simulink model "system2020b"  (R2020b)
settings: Solver=VariableStepAuto  StartTime=0.0  StopTime=50  RelTol=1e-3
InitFcn:
  | parametriEgo
values from neighbouring files (symbols this model uses):
  campnormalized = campmag/sqrt(campmag(1)^2+campmag(2)^2+campmag(3)^2)    [parametriEgo.m]
  g = 9.81    [kalman_jacobian.m]    (also in parametriEgo.m = [0; 0; -9.81])
  initial_conditions = [0,0,0*pi/180,0*pi/180,0,0]    [parametriEgo.m]
  k_e_qf = 0.1    [ego_control_gains_sensors.m]
  ki_e_nu_speed = 2.5    [ego_control_gains_sensors.m]
  kp_e_nu_phidot = 7    [ego_control_gains_sensors.m]
  kp_e_nu_speed = 6    [ego_control_gains_sensors.m]
  kp_e_nu_thetadot = 7    [ego_control_gains_sensors.m]
  kp_e_theta = 40    [ego_control_gains_sensors.m]
  l = 0.248    [parametriEgo.m]
  L = 0.379    [parametriEgo.m]
  mb = 21.7+0.536*10+0.381*2    (= 27.822)    [parametriEgo.m]
  mw = 1.6    [parametriEgo.m]
  P0 = 1500*eye(7)    [parametriEgo.m]
  r = 0.13    [parametriEgo.m]
  seedAcc1 = ceil(rand()*10)    [parametriEgo.m]
  seedAcc2 = ceil(rand()*10)    [parametriEgo.m]
  seedGyro1 = ceil(rand()*10)    [parametriEgo.m]
  seedGyro2 = ceil(rand()*10)    [parametriEgo.m]
  tau_max = 11    [parametriEgo.m]
  totAccNoisePower = (accNoiseDens* 10^-6 * 9.8)^2    (= 8.6436e-06)    [parametriEgo.m]
  totGyroNoisePower = (gyroNoiseDens * pi/180)^2    (= 3.04617419787e-06)    [parametriEgo.m]
  Ts = 1/100    (= 0.01)    [parametriEgo.m]
  TsController = 1/100    (= 0.01)    [parametriEgo.m]
  TsGraph = 1/100    (= 0.01)    [parametriEgo.m]
  x0 = zeros(7,1)    [parametriEgo.m]
undefined symbols (not defined in the file or in its folder): alpha
libraries: simulink_extras x45, simulink x10, eeGeneralControl x3
(part 1 of 3)
settings Model: Creator=pcfilm  LastModifiedBy=stefa
settings DebuggingCC: SFMachineParentedDataDiag=error

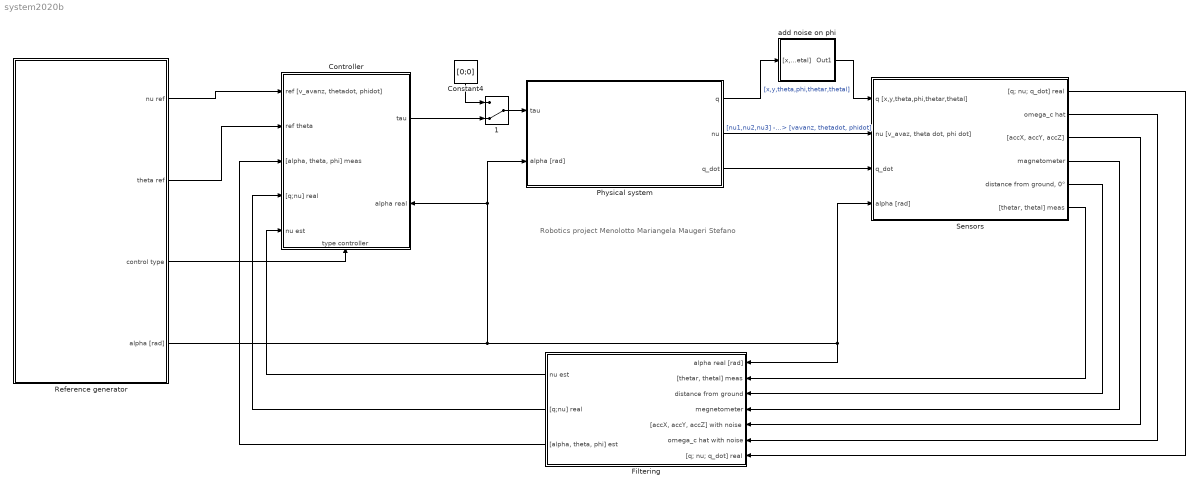
== system system2020b ==
  note: Robotics project
      | Menolotto Mariangela
      | Maugeri Stefano
  " 1" : ManualSwitch  StopFcn=show_results  CurrentSetting=0
  Constant4 : Constant  Value=[0;0]  SampleTime=-1
  Controller : Subsystem
      settings: PortSchema="{\"entries\":[{\"content\":{\"sides\":[{\"content\":{\"connectorIds\":[\"In1\",\"In2\",\"In3\",\"In4\",\"In5\"]},\"type\":\"ConnectorPlacement.EquallySpacedRectSide\",\"uuid\":\"8f36a280-abce-482b-9b97-e189d55cf96d\"},{\"content\":{\"connectorIds\":[\"Out1\",\"In7\"],\"side\":\"RIGHT\"},\"type\":\"ConnectorPlacement.EquallySpacedRectSide\",\"uuid\":\"71f54387-a45a-4e5e-9582-a0f1ed7853f2\"},{\"content\":{\"connectorIds\":[],\"side\":\"TOP\"},\"type\":\"ConnectorPlacement.EquallySpacedRectSide\",\"uuid\":\"bc3039b8-0052-42d5-8d22-75d00eb9e222\"},{\"content\":{\"connectorIds\":[\"In6\"],\"side\":\"BOTTOM\"},\"type\":\"ConnectorPlacement.EquallySpacedRectSide\",\"uuid\":\"65646135-8cf5-4f6c-bd6c-0ad1be6a71b3\"}]},\"type\":\"ConnectorPlacement.EquallySpacedConnector\",\"uuid\":\"29576908-5cc3-45a2-91a3-f3615a274226\"}],\"packageUris\":[\"http://schema.mathworks.com/mf0/Connector/R2020b\"],\"version\":\"1.0\"}"
  Filtering : Subsystem
  Physical system : Subsystem
  Reference generator : Subsystem
  Sensors : Subsystem
  add noise on phi : Subsystem
  wires:
  Constant4/1 -> " 1"/1
  Controller/1(tau) -> " 1"/2
  Physical system/2(nu) -> Sensors/2("nu [v_avaz, theta dot, phi dot]")  "[nu1,nu2,nu3] -> [vavanz, thetadot, phidot]"
  " 1"/1 -> Physical system/1(tau)
  Reference generator/3(control type) -> Controller/6(type controller)
  Reference generator/1(nu ref) -> Controller/1("ref [v_avanz, thetadot, phidot]")
  Reference generator/2(theta ref) -> Controller/2(ref theta)
  Reference generator/4(alpha [rad]) -> Physical system/2(alpha [rad]), Controller/7(alpha real), Sensors/4(alpha [rad]), Filtering/1(alpha real [rad])
  Sensors/2(omega_c hat) -> Filtering/6(omega_c hat with noise)
  Sensors/3("[accX, accY, accZ]") -> Filtering/5("[accX, accY, accZ] with noise")
  Sensors/1("[q; nu; q_dot] real") -> Filtering/7("[q; nu; q_dot] real")
  Filtering/1(nu est) -> Controller/5(nu est)
  Physical system/3(q_dot) -> Sensors/3(q_dot)
  Filtering/2("[q;nu] real") -> Controller/4("[q;nu] real")
  Sensors/4(magnetometer) -> Filtering/4(megnetometer)
  Filtering/3("[alpha, theta, phi] est") -> Controller/3("[alpha, theta, phi] meas")
  Sensors/5("distance from ground, 0°") -> Filtering/3(distance from ground)
  Physical system/1(q) -> add noise on phi/1("[x,y,theta,phi,thetar,thetal]")  "[x,y,theta,phi,thetar,thetal]"
  add noise on phi/1(Out1) -> Sensors/1(q [x,y,theta,phi,thetar,thetal])
  Sensors/6("[thetar, thetal] meas") -> Filtering/2("[thetar, thetal] meas")

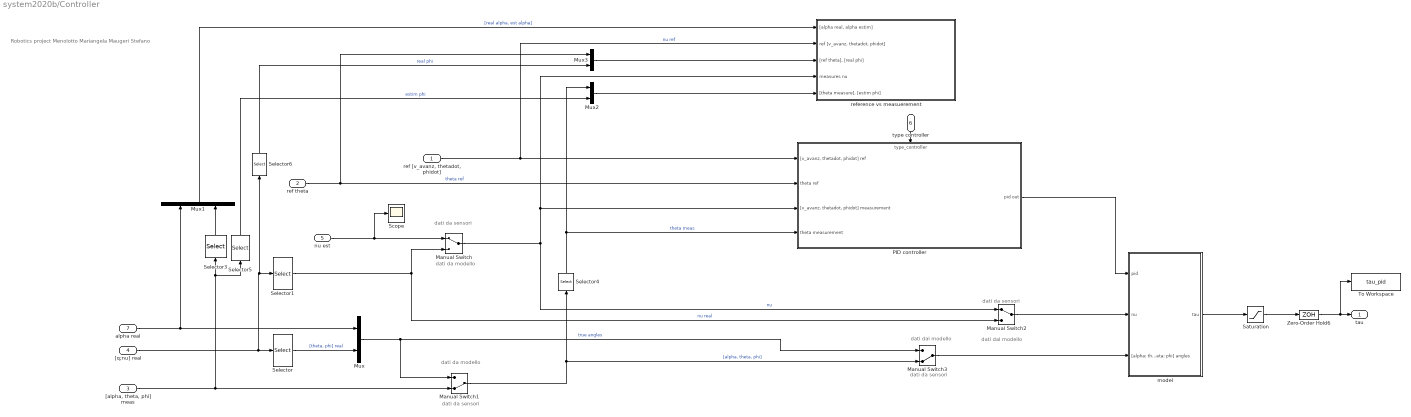
== system system2020b/Controller ==
  note: dati dal modello
  note: dati da sensori
  note: dati da modello
  note: dati da modello
  note: dati da sensori
  note: dati dal modello
  note: dati da sensori
  note: dati da sensori
  note: Robotics project
      | Menolotto Mariangela
      | Maugeri Stefano
  "ref [v_avanz, thetadot, phidot]" : Inport
  ref theta : Inport  Port=2
  "[alpha, theta, phi] meas" : Inport  Port=3
  "[q;nu] real" : Inport  Port=4
  nu est : Inport  Port=5
  type controller : Inport  Port=6
  alpha real : Inport  Port=7
  Manual Switch : ManualSwitch
  Manual Switch1 : ManualSwitch  CurrentSetting=0
  Manual Switch2 : ManualSwitch
  Manual Switch3 : ManualSwitch  CurrentSetting=0
  Mux{,1..3} (4 alike) : Mux  Inputs=2
  PID controller : Subsystem
      settings: PortSchema="{\"entries\":[{\"content\":{\"sides\":[{\"content\":{\"connectorIds\":[\"In1\",\"In2\",\"In3\",\"In4\"]},\"type\":\"ConnectorPlacement.EquallySpacedRectSide\",\"uuid\":\"d9cb11f3-1c4d-43fe-a12d-5969826cc334\"},{\"content\":{\"connectorIds\":[\"Out1\"],\"side\":\"RIGHT\"},\"type\":\"ConnectorPlacement.EquallySpacedRectSide\",\"uuid\":\"ad772aa2-2e51-4343-aa11-c9e8da0a1620\"},{\"content\":{\"connectorIds\":[\"In5\"],\"side\":\"TOP\"},\"type\":\"ConnectorPlacement.EquallySpacedRectSide\",\"uuid\":\"78560075-815c-4832-b262-2927709ef249\"},{\"content\":{\"connectorIds\":[],\"side\":\"HIDDEN\"},\"type\":\"ConnectorPlacement.EquallySpacedRectSide\",\"uuid\":\"b300515a-818b-474a-87d6-584e57c75196\"}]},\"type\":\"ConnectorPlacement.EquallySpacedConnector\",\"uuid\":\"c875b1c4-dcf7-4b75-8d7e-da3564072335\"}],\"packageUris\":[\"http://schema.mathworks.com/mf0/Connector/R2020b\"],\"version\":\"1.0\"}"
  Saturation : Saturate  UpperLimit=tau_max  LowerLimit=-tau_max
  Scope : Scope
  Selector : Selector  InputPortWidth=9  IndexOptions=Index vector (dialog)  Indices=[3 4]  OutputSizes=1
  Selector1 : Selector  InputPortWidth=9  IndexOptions=Index vector (dialog)  Indices=[7 8 9]  OutputSizes=1
  Selector3 : Selector  InputPortWidth=3  IndexOptions=Index vector (dialog)  Indices=1  OutputSizes=1
  Selector4 : Selector  InputPortWidth=3  IndexOptions=Index vector (dialog)  Indices=2  OutputSizes=1
  Selector5 : Selector  InputPortWidth=3  IndexOptions=Index vector (dialog)  Indices=3  OutputSizes=1
  Selector6 : Selector  InputPortWidth=9  IndexOptions=Index vector (dialog)  Indices=4  OutputSizes=1
  To Workspace : ToWorkspace  VariableName=tau_pid  SampleTime=-1
      settings: MaxDataPoints=1
  Zero-Order Hold6 : ZeroOrderHold  SampleTime=TsController
  model : Subsystem
  reference vs measuerement : Subsystem
  tau : Outport
  wires:
  Saturation/1 -> Zero-Order Hold6/1
  Manual Switch/1 -> PID controller/3("[v_avanz, thetadot, phidot] measurement"), reference vs measuerement/4(measures nu), Manual Switch2/1  "nu"
  model/1(tau) -> Saturation/1
  type controller/1 -> PID controller/5(type_controller)
  "ref [v_avanz, thetadot, phidot]"/1 -> PID controller/1("[v_avanz, thetadot, phidot] ref"), reference vs measuerement/2("ref [v_avanz, thetadot, phidot]")  "nu ref"
  ref theta/1 -> PID controller/2(theta ref), Mux3/1  "theta ref"
  PID controller/1(pid out) -> model/1(pid)
  Manual Switch1/1 -> Manual Switch3/2, Selector4/1  "[alpha, theta, phi]"
  Selector4/1 -> PID controller/4(theta measurement), Mux2/1  "theta meas"
  nu est/1 -> Scope/1, Manual Switch/1
  "[q;nu] real"/1 -> Selector/1, Selector1/1, Selector6/1
  "[alpha, theta, phi] meas"/1 -> Selector5/1, Selector3/1, Manual Switch1/2
  alpha real/1 -> Mux1/1, Mux/1
  Selector/1 -> Mux/2  "[theta, phi] real"
  Mux/1 -> Manual Switch3/1, Manual Switch1/1  "true angles"
  Selector1/1 -> Manual Switch2/2, Manual Switch/2  "nu real"
  Selector3/1 -> Mux1/2
  Mux1/1 -> reference vs measuerement/1("[alpha real, alpha estim]")  "[real alpha, est alpha]"
  Manual Switch2/1 -> model/2(nu)
  Manual Switch3/1 -> model/3("[alpha; theta; phi] angles")
  Mux3/1 -> reference vs measuerement/3("[ref theta], [real phi]")
  Mux2/1 -> reference vs measuerement/5("[theta measure], [estim phi]")
  Selector6/1 -> Mux3/2  "real phi"
  Selector5/1 -> Mux2/2  "estim phi"
  Zero-Order Hold6/1 -> To Workspace/1, tau/1

== system system2020b/Filtering ==
  note: estimate angles from mahony
  note: estimate angles from kalman
  note: Robotics project
      | Menolotto Mariangela
      | Maugeri Stefano
  alpha real [rad] : Inport
  "[thetar, thetal] meas" : Inport  Port=2
  distance from ground : Inport  Port=3
  megnetometer : Inport  Port=4
  "[accX, accY, accZ] with noise" : Inport  Port=5
  omega_c hat with noise : Inport  Port=6
  "[q; nu; q_dot] real" : Inport  Port=7
  Clock : Clock
  Demux : Demux  Outputs=[3, 3, 9]
  Kalman filter : Subsystem
  Mahony + distance sensor : Subsystem
  Mux : Mux  Inputs=[3, 3, 9]
  Mux1 : Mux  Inputs=[3, 3, 9]
  Switch : Switch  Criteria=u2 > Threshold  Threshold=0.8
  Zero-Order Hold5 : ZeroOrderHold  SampleTime=Ts
  mux signals : Subsystem
  real signals vs estimate signals : Subsystem
  real signals vs kalman estimation vs mahony estimation : Subsystem
  nu est : Outport
  "[q;nu] real" : Outport  Port=2
  "[alpha, theta, phi] est" : Outport  Port=3
  wires:
  "[q; nu; q_dot] real"/1 -> mux signals/1("[q; nu; q_dot] real")
  mux signals/2("[q;nu]") -> Mux1/3, Mux/3
  alpha real [rad]/1 -> real signals vs estimate signals/4(real alpha), real signals vs kalman estimation vs mahony estimation/3(alpha real1)
  Mux/1 -> real signals vs kalman estimation vs mahony estimation/1(data from mahony), Switch/3  "mahony data"
  distance from ground/1 -> Mahony + distance sensor/1(d)
  "[accX, accY, accZ] with noise"/1 -> Mahony + distance sensor/2("[accX, accY, accZ] with noise"), Kalman filter/3("[accX, accY, accZ] with noise")
  omega_c hat with noise/1 -> Mahony + distance sensor/3(omega_c), Kalman filter/4(omega_c)
  megnetometer/1 -> Kalman filter/5(magnetometer), Mahony + distance sensor/4(magnetomiter)
  mux signals/1(v_forward) -> Kalman filter/2(v forward), Mahony + distance sensor/5(v forward)
  Mahony + distance sensor/1("[v_avanz real, thetadot, phidot] est") -> Mux/1
  Mahony + distance sensor/2("[alpha theta phi] est") -> Mux/2
  Switch/1 -> Demux/1
  Kalman filter/2("[alpha theta phi] est") -> Mux1/2
  Kalman filter/1("[v_forward, thetadot, phidot] est") -> Mux1/1
  Mux1/1 -> real signals vs kalman estimation vs mahony estimation/2(data from kalman), Switch/1  "kalman data"
  Demux/1 -> nu est/1, real signals vs estimate signals/1(nu est)
  Demux/2 -> "[alpha, theta, phi] est"/1, real signals vs estimate signals/2("[alpha, theta, phi] est")
  Demux/3 -> real signals vs estimate signals/3("[q;nu] real"), "[q;nu] real"/1
  "[thetar, thetal] meas"/1 -> Kalman filter/1("[thetar, thetal] meas")
  Clock/1 -> Zero-Order Hold5/1
  Zero-Order Hold5/1 -> Switch/2

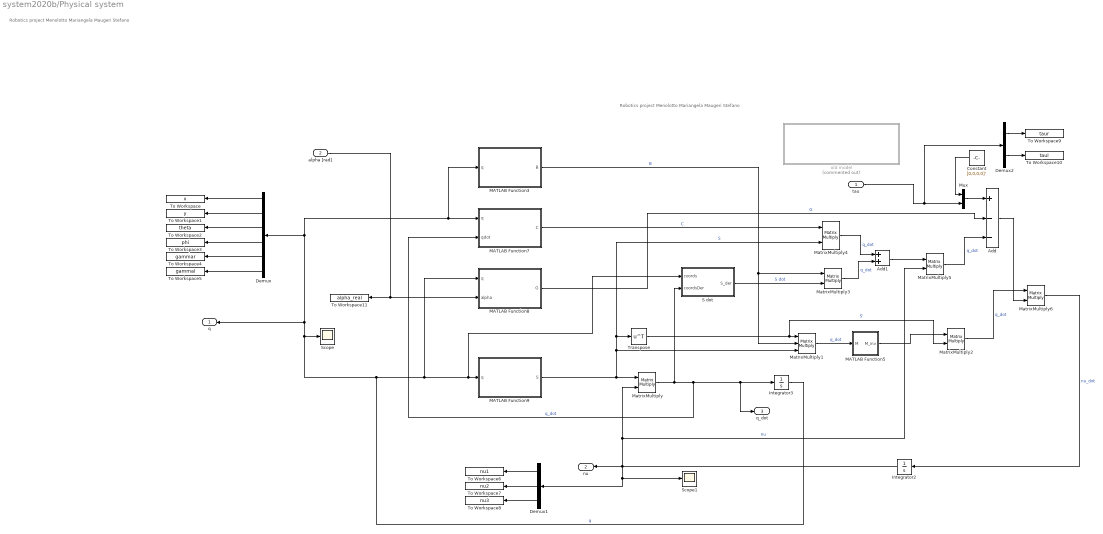
== system system2020b/Physical system ==
  note: Robotics project
      | Menolotto Mariangela
      | Maugeri Stefano
  note: Robotics project
      | Menolotto Mariangela
      | Maugeri Stefano
  tau : Inport
  alpha [rad] : Inport  Port=2
  Add : Sum  Inputs=+--
  Add1 : Sum
  Constant : Constant  Value=[0,0,0,0]'  SampleTime=-1
  Demux : Demux  Outputs=6
  Demux1 : Demux  Outputs=3
  Demux2 : Demux  Outputs=2
  Integrator2 : Integrator  InitialCondition=[0; 0; 0]
  Integrator3 : Integrator  InitialCondition=initial_conditions
  MATLAB Function3 : MATLAB Function  TreatAsAtomicUnit=on
  MATLAB Function5 : MATLAB Function  TreatAsAtomicUnit=on
  MATLAB Function7 : MATLAB Function  TreatAsAtomicUnit=on
  MATLAB Function8 : MATLAB Function  TreatAsAtomicUnit=on
  MATLAB Function9 : MATLAB Function  TreatAsAtomicUnit=on
  MatrixMultiply{,2..6} (6 alike) : Product  Multiplication=Matrix(*)
  MatrixMultiply1 : Product  Inputs=3  Multiplication=Matrix(*)
  Mux : Mux  Inputs=2
  S dot : MATLAB Function  TreatAsAtomicUnit=on
  Scope : Scope
  Scope1 : Scope
  To Workspace : ToWorkspace  VariableName=x  SaveFormat=Timeseries  SampleTime=TsGraph
  To Workspace1 : ToWorkspace  VariableName=y  SaveFormat=Timeseries  SampleTime=TsGraph
  To Workspace10 : ToWorkspace  VariableName=taul  SaveFormat=Timeseries  SampleTime=TsGraph
  To Workspace11 : ToWorkspace  VariableName=alpha_real  SaveFormat=Timeseries  SampleTime=TsGraph
  To Workspace2 : ToWorkspace  VariableName=theta  SaveFormat=Timeseries  SampleTime=TsGraph
  To Workspace3 : ToWorkspace  VariableName=phi  SaveFormat=Timeseries  SampleTime=TsGraph
  To Workspace4 : ToWorkspace  VariableName=gammar  SaveFormat=Timeseries  SampleTime=TsGraph
  To Workspace5 : ToWorkspace  VariableName=gammal  SaveFormat=Timeseries  SampleTime=TsGraph
  To Workspace6 : ToWorkspace  VariableName=nu1  SaveFormat=Timeseries  SampleTime=TsGraph
  To Workspace7 : ToWorkspace  VariableName=nu2  SaveFormat=Timeseries  SampleTime=TsGraph
  To Workspace8 : ToWorkspace  VariableName=nu3  SaveFormat=Timeseries  SampleTime=TsGraph
  To Workspace9 : ToWorkspace  VariableName=taur  SaveFormat=Timeseries  SampleTime=TsGraph
  Transpose : Math  Operator=transpose  SaturateOnIntegerOverflow=on
  old model : Subsystem  Commented=on
  q : Outport
  nu : Outport  Port=2
  q_dot : Outport  Port=3
  wires:
  MATLAB Function9/1(S) -> MatrixMultiply1/3, Transpose/1, MatrixMultiply4/2, MatrixMultiply/1  "S"
  Integrator3/1 -> Scope/1, MATLAB Function3/1(q), MATLAB Function7/1(q), Demux/1, q/1, MATLAB Function8/1(q), MATLAB Function9/1(q), S dot/1(coords)  "q"
  S dot/1(S_der) -> MatrixMultiply3/2  "S dot"
  MATLAB Function3/1(B) -> MatrixMultiply3/1, MatrixMultiply1/2  "B"
  Integrator2/1 -> Demux1/1, Scope1/1, MatrixMultiply5/2, MatrixMultiply/2, nu/1  "nu"
  MATLAB Function8/1(G) -> Add/2  "G"
  Transpose/1 -> MatrixMultiply2/2, MatrixMultiply1/1  "S'"
  MatrixMultiply1/1 -> MATLAB Function5/1(M)  "q_dot"
  MatrixMultiply3/1 -> Add1/2  "q_dot"
  MatrixMultiply/1 -> MATLAB Function7/2(qdot), q_dot/1, Integrator3/1, S dot/2(coordsDer)  "q_dot"
  MATLAB Function7/1(C) -> MatrixMultiply4/1  "C"
  Add1/1 -> MatrixMultiply5/1
  MatrixMultiply4/1 -> Add1/1  "q_dot"
  MatrixMultiply5/1 -> Add/3  "q_dot"
  Add/1 -> MatrixMultiply6/2
  MatrixMultiply6/1 -> Integrator2/1  "nu_dot"
  MATLAB Function5/1(M_inv) -> MatrixMultiply2/1
  MatrixMultiply2/1 -> MatrixMultiply6/1  "q_dot"
  Demux/5 -> To Workspace4/1
  Demux/2 -> To Workspace1/1
  Demux/6 -> To Workspace5/1
  Mux/1 -> Add/1
  Constant/1 -> Mux/1
  Demux1/1 -> To Workspace6/1
  Demux1/2 -> To Workspace7/1
  Demux1/3 -> To Workspace8/1
  tau/1 -> Demux2/1, Mux/2
  Demux2/1 -> To Workspace9/1
  Demux2/2 -> To Workspace10/1
  alpha [rad]/1 -> To Workspace11/1, MATLAB Function8/2(alpha)
  Demux/4 -> To Workspace3/1
  Demux/3 -> To Workspace2/1
  Demux/1 -> To Workspace/1

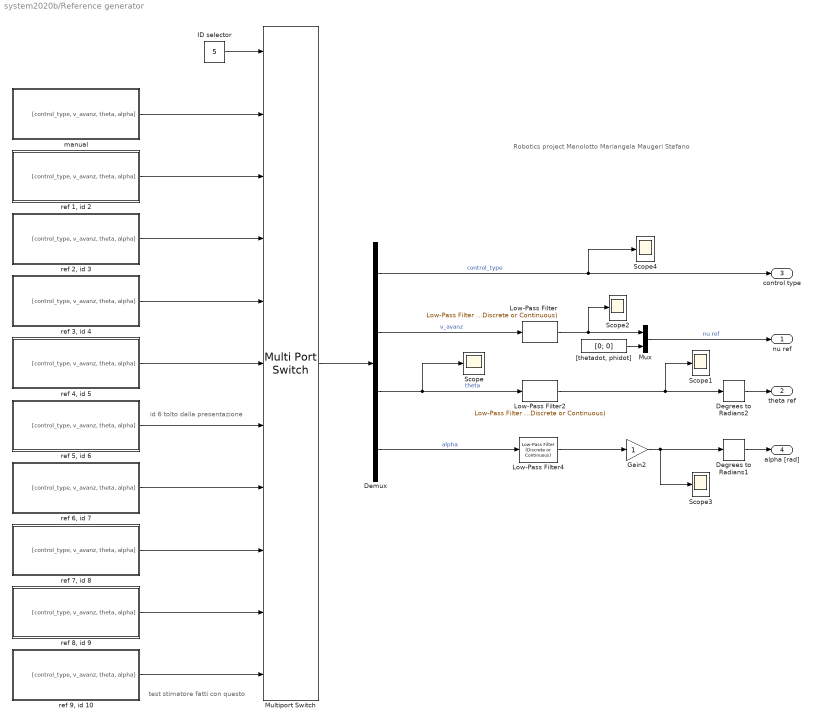
== system system2020b/Reference generator ==
  note: test stimatore fatti con questo
  note: id 6 tolto dalla presentazione
  note: Robotics project
      | Menolotto Mariangela
      | Maugeri Stefano
  Degrees to Radians1 : simulink_extras/Transformations/Degrees to Radians
  Degrees to Radians2 : simulink_extras/Transformations/Degrees to Radians
  Demux : Demux
  Gain2 : Gain
  ID selector : Constant  Value=5
  Low-Pass Filter : eeGeneralControl/Low-Pass Filter (Discrete or Continuous)  K=1  T=1  B=inf  A=-inf  init_option=Inherited from block input  x0=0  Ts=-1
  Low-Pass Filter2 : eeGeneralControl/Low-Pass Filter (Discrete or Continuous)  K=1  T=5  B=inf  A=-inf  init_option=Inherited from block input  x0=0  Ts=-1
  Low-Pass Filter4 : eeGeneralControl/Low-Pass Filter (Discrete or Continuous)  K=1  T=1  B=inf  A=-inf  init_option=Inherited from block input  x0=0  Ts=-1
  Multiport Switch : MultiPortSwitch  Inputs=10
  Mux : Mux  Inputs=2
  Scope{,1..4} (5 alike) : Scope
  "[thetadot, phidot]" : Constant  Value=[0; 0]
  manual : Subsystem
  "ref 1, id 2" : Subsystem
  "ref 2, id 3" : Subsystem
  "ref 3, id 4" : Subsystem
  "ref 4, id 5" : Subsystem
  "ref 5, id 6" : Subsystem
  "ref 6, id 7" : Subsystem
  "ref 7, id 8" : Subsystem
  "ref 8, id 9" : Subsystem
  "ref 9, id 10" : Subsystem
  nu ref : Outport
  theta ref : Outport  Port=2
  control type : Outport  Port=3
  alpha [rad] : Outport  Port=4
  wires:
  "[thetadot, phidot]"/1 -> Mux/2
  Mux/1 -> nu ref/1  "nu ref"
  Degrees to Radians1/1 -> alpha [rad]/1
  Low-Pass Filter2/1 -> Scope1/1, Degrees to Radians2/1
  Low-Pass Filter/1 -> Scope2/1, Mux/1
  Low-Pass Filter4/1 -> Gain2/1
  Gain2/1 -> Scope3/1, Degrees to Radians1/1
  Demux/4 -> Low-Pass Filter4/1  "alpha"
  Demux/1 -> Scope4/1, control type/1  "control_type"
  Demux/2 -> Low-Pass Filter/1  "v_avanz"
  Demux/3 -> Scope/1, Low-Pass Filter2/1  "theta"
  Multiport Switch/1 -> Demux/1
  manual/1("[control_type, v_avanz, theta, alpha]") -> Multiport Switch/2
  ID selector/1 -> Multiport Switch/1
  "ref 1, id 2"/1("[control_type, v_avanz, theta, alpha]") -> Multiport Switch/3
  "ref 2, id 3"/1("[control_type, v_avanz, theta, alpha]") -> Multiport Switch/4
  "ref 3, id 4"/1("[control_type, v_avanz, theta, alpha]") -> Multiport Switch/5
  Degrees to Radians2/1 -> theta ref/1
  "ref 4, id 5"/1("[control_type, v_avanz, theta, alpha]") -> Multiport Switch/6
  "ref 5, id 6"/1("[control_type, v_avanz, theta, alpha]") -> Multiport Switch/7
  "ref 6, id 7"/1("[control_type, v_avanz, theta, alpha]") -> Multiport Switch/8
  "ref 7, id 8"/1("[control_type, v_avanz, theta, alpha]") -> Multiport Switch/9
  "ref 8, id 9"/1("[control_type, v_avanz, theta, alpha]") -> Multiport Switch/10
  "ref 9, id 10"/1("[control_type, v_avanz, theta, alpha]") -> Multiport Switch/11

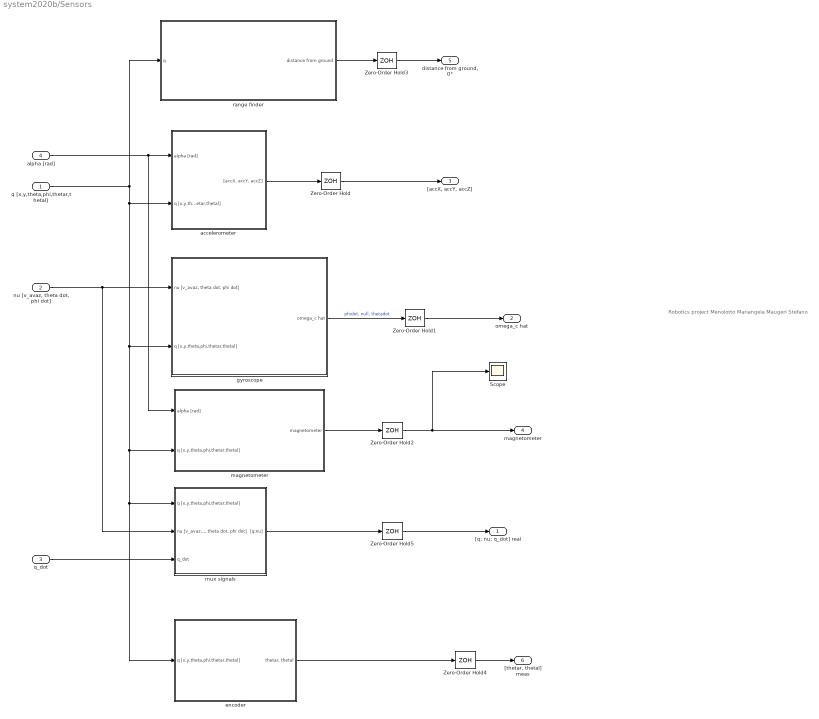
== system system2020b/Sensors ==
  note: Robotics project
      | Menolotto Mariangela
      | Maugeri Stefano
  q [x,y,theta,phi,thetar,thetal] : Inport
  "nu [v_avaz, theta dot, phi dot]" : Inport  Port=2
  q_dot : Inport  Port=3
  alpha [rad] : Inport  Port=4
  Scope : Scope
  Zero-Order Hold{,1..5} (6 alike) : ZeroOrderHold  SampleTime=Ts
  accelerometer : Subsystem
  encoder : Subsystem
  gyroscope : Subsystem
  "magnetometer   " : Subsystem
  mux signals : Subsystem
  range finder : Subsystem
  "[q; nu; q_dot] real" : Outport
  omega_c hat : Outport  Port=2
  "[accX, accY, accZ]" : Outport  Port=3
  magnetometer : Outport  Port=4
  "distance from ground, 0°" : Outport  Port=5
  "[thetar, thetal] meas" : Outport  Port=6
  wires:
  "nu [v_avaz, theta dot, phi dot]"/1 -> mux signals/2("nu [v_avaz, theta dot, phi dot]"), gyroscope/1("nu [v_avaz, theta dot, phi dot]")
  q [x,y,theta,phi,thetar,thetal]/1 -> gyroscope/2(q [x,y,theta,phi,thetar,thetal]), "magnetometer   "/2(q [x,y,theta,phi,thetar,thetal]), encoder/1(q [x,y,theta,phi,thetar,thetal]), mux signals/1(q [x,y,theta,phi,thetar,thetal]), accelerometer/2(q [x,y,theta,phi,thetar,thetal]), range finder/1(q)
  accelerometer/1("[accX, accY, accZ]") -> Zero-Order Hold/1
  gyroscope/1(omega_c hat) -> Zero-Order Hold1/1  "phidot, null, thetadot"
  Zero-Order Hold/1 -> "[accX, accY, accZ]"/1
  Zero-Order Hold1/1 -> omega_c hat/1
  mux signals/1("[q;nu]") -> Zero-Order Hold5/1
  q_dot/1 -> mux signals/3(q_dot)
  alpha [rad]/1 -> "magnetometer   "/1(alpha [rad]), accelerometer/1(alpha [rad])
  "magnetometer   "/1(magnetometer) -> Zero-Order Hold2/1
  Zero-Order Hold2/1 -> Scope/1, magnetometer/1
  range finder/1(distance from ground) -> Zero-Order Hold3/1
  Zero-Order Hold3/1 -> "distance from ground, 0°"/1
  encoder/1("thetar, thetal") -> Zero-Order Hold4/1
  Zero-Order Hold4/1 -> "[thetar, thetal] meas"/1
  Zero-Order Hold5/1 -> "[q; nu; q_dot] real"/1

== system system2020b/add noise on phi ==
  note: Robotics project
      | Menolotto Mariangela
      | Maugeri Stefano
  "[x,y,theta,phi,thetar,thetal]" : Inport
  Degrees to Radians : simulink_extras/Transformations/Degrees to Radians
  Mux : Mux  Inputs=3
  Product : Product
  Radians to Degrees2 : simulink_extras/Transformations/Radians to Degrees
  Random Number : RandomNumber  Variance=3  SampleTime=0.1
  Scope : Scope  NumInputPorts=2
  Selector1 : Selector  InputPortWidth=6  IndexOptions=Index vector (dialog)  Indices=4  OutputSizes=1
  Selector2 : Selector  InputPortWidth=6  IndexOptions=Index vector (dialog)  Indices=[1 2 3]  OutputSizes=1
  Selector3 : Selector  InputPortWidth=6  IndexOptions=Index vector (dialog)  Indices=[5 6]  OutputSizes=1
  Step : Step  Time=20  After=0  SampleTime=0
  Sum : Sum  Inputs=++|
  Out1 : Outport
  wires:
  Sum/1 -> Degrees to Radians/1, Scope/2
  "[x,y,theta,phi,thetar,thetal]"/1 -> Out1/1, Selector3/1, Selector1/1, Selector2/1
  Product/1 -> Sum/1
  Degrees to Radians/1 -> Mux/2
  Step/1 -> Product/2
  Radians to Degrees2/1 -> Scope/1, Sum/2
  Selector3/1 -> Mux/3
  Random Number/1 -> Product/1
  Selector1/1 -> Radians to Degrees2/1
  Mux/1 -> ?
  Selector2/1 -> Mux/1

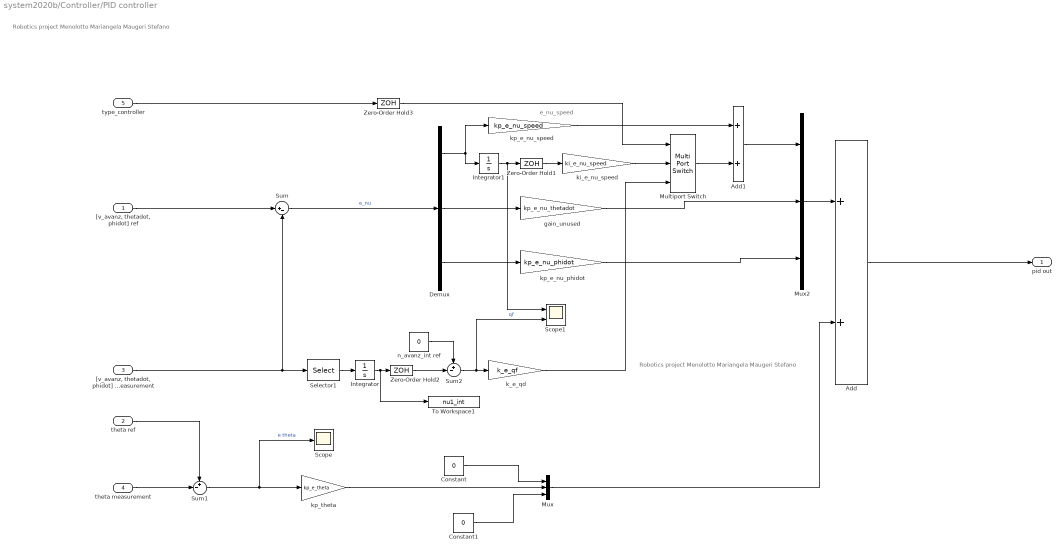
== system system2020b/Controller/PID controller ==
  note: e_nu_speed
  note: Robotics project
      | Menolotto Mariangela
      | Maugeri Stefano
  note: Robotics project
      | Menolotto Mariangela
      | Maugeri Stefano
  "[v_avanz, thetadot, phidot] ref" : Inport
  theta ref : Inport  Port=2
  "[v_avanz, thetadot, phidot] measurement" : Inport  Port=3
  theta measurement : Inport  Port=4
  type_controller : Inport  Port=5
  Add : Sum
  Add1 : Sum
  Constant : Constant  Value=0  SampleTime=-1
  Constant1 : Constant  Value=0  SampleTime=-1
  Demux : Demux  Outputs=3
  Integrator : Integrator
  Integrator1 : Integrator
  Multiport Switch : MultiPortSwitch  Inputs=2
  Mux : Mux  Inputs=3
  Mux2 : Mux  Inputs=3
  Scope : Scope
  Scope1 : Scope  NumInputPorts=2
  Selector1 : Selector  InputPortWidth=3  IndexOptions=Index vector (dialog)  Indices=[1]  OutputSizes=1
  Sum : Sum  Inputs=|+-
  Sum1 : Sum  Inputs=+-|
  Sum2 : Sum  Inputs=+-|
  To Workspace1 : ToWorkspace  VariableName=nu1_int  SaveFormat=Timeseries  SampleTime=TsGraph
  Zero-Order Hold1 : ZeroOrderHold  SampleTime=TsController
  Zero-Order Hold2 : ZeroOrderHold  SampleTime=TsController
  Zero-Order Hold3 : ZeroOrderHold  SampleTime=TsController
  gain_unused : Gain  Gain=kp_e_nu_thetadot
  k_e_qd : Gain  Gain=k_e_qf
  ki_e_nu_speed : Gain  Gain=ki_e_nu_speed
  kp_e_nu_phidot : Gain  Gain=kp_e_nu_phidot
  kp_e_nu_speed : Gain  Gain=kp_e_nu_speed
  kp_theta : Gain  Gain=kp_e_theta
  n_avanz_int ref : Constant  Value=0  SampleTime=Ts
  pid out : Outport
  wires:
  Integrator/1 -> Zero-Order Hold2/1, To Workspace1/1
  kp_e_nu_speed/1 -> Add1/1
  gain_unused/1 -> Mux2/2
  "[v_avanz, thetadot, phidot] measurement"/1 -> Sum/2, Selector1/1
  kp_e_nu_phidot/1 -> Mux2/3
  Demux/2 -> gain_unused/1
  Multiport Switch/1 -> Add1/2
  Demux/3 -> kp_e_nu_phidot/1
  Mux2/1 -> Add/1
  Constant1/1 -> Mux/3
  n_avanz_int ref/1 -> Sum2/1
  Demux/1 -> kp_e_nu_speed/1, Integrator1/1
  Selector1/1 -> Integrator/1
  "[v_avanz, thetadot, phidot] ref"/1 -> Sum/1
  Sum2/1 -> Scope1/2, k_e_qd/1  "qf"
  Constant/1 -> Mux/1
  Sum1/1 -> Scope/1, kp_theta/1  "e theta"
  Sum/1 -> Demux/1  "e_nu"
  theta ref/1 -> Sum1/1
  type_controller/1 -> Zero-Order Hold3/1
  theta measurement/1 -> Sum1/2
  Integrator1/1 -> Zero-Order Hold1/1, Scope1/1
  Mux/1 -> Add/2
  k_e_qd/1 -> Multiport Switch/3
  Add/1 -> pid out/1
  kp_theta/1 -> Mux/2
  ki_e_nu_speed/1 -> Multiport Switch/2
  Add1/1 -> Mux2/1
  Zero-Order Hold1/1 -> ki_e_nu_speed/1
  Zero-Order Hold2/1 -> Sum2/2
  Zero-Order Hold3/1 -> Multiport Switch/1

== system system2020b/Controller/model ==
  note: Robotics project
      | Menolotto Mariangela
      | Maugeri Stefano
  pid : Inport
  nu : Inport  Port=2
  "[alpha; theta; phi] angles" : Inport  Port=3
  Add1 : Sum
  Add2 : Sum  Inputs=+++
  MATLAB Function1 : MATLAB Function  TreatAsAtomicUnit=on
  MATLAB Function2 : MATLAB Function  TreatAsAtomicUnit=on
  MATLAB Function3 : MATLAB Function  TreatAsAtomicUnit=on
  MATLAB Function7 : MATLAB Function  TreatAsAtomicUnit=on
  MATLAB Function8 : MATLAB Function  TreatAsAtomicUnit=on
  MATLAB Function9 : MATLAB Function  TreatAsAtomicUnit=on
  MatrixMultiply : Product  Inputs=3  Multiplication=Matrix(*)
  MatrixMultiply1 : Product  Multiplication=Matrix(*)
  MatrixMultiply2 : Product  Multiplication=Matrix(*)
  MatrixMultiply3 : Product  Inputs=3  Multiplication=Matrix(*)
  MatrixMultiply4 : Product  Inputs=3  Multiplication=Matrix(*)
  MatrixMultiply5 : Product  Multiplication=Matrix(*)
  S dot : MATLAB Function  TreatAsAtomicUnit=on
  Selector : Selector  InputPortWidth=3  IndexOptions=Index vector (dialog)  Indices=[2 3]  OutputSizes=1
  Transpose : Math  Operator=transpose  SaturateOnIntegerOverflow=on
  get nu_acc : Selector  InputPortWidth=3  IndexOptions=Index vector (dialog)  Indices=[2 3]  OutputSizes=1
  tau : Outport
  wires:
  Selector/1 -> MatrixMultiply5/2
  MATLAB Function2/1(Sr_inv) -> MatrixMultiply5/1  "S"
  MatrixMultiply5/1 -> tau/1
  "[alpha; theta; phi] angles"/1 -> MATLAB Function9/1(angles), MATLAB Function3/1(angles), MATLAB Function1/1(angles), S dot/1(angles), MATLAB Function8/1(angles), MATLAB Function7/1(angles)
  MatrixMultiply2/1 -> Add1/2
  MatrixMultiply3/1 -> Add2/1
  Add2/1 -> MatrixMultiply2/2
  MatrixMultiply4/1 -> Add2/2
  MatrixMultiply/1 -> MatrixMultiply1/1
  Add1/1 -> Selector/1
  get nu_acc/1 -> S dot/2(nu_acc), MATLAB Function7/2(nu_acc)
  S dot/1(S_der) -> MatrixMultiply3/2  "S dot"
  MatrixMultiply1/1 -> Add1/1
  MATLAB Function3/1(B) -> MatrixMultiply/2, MatrixMultiply3/1  "B"
  MATLAB Function7/1(C) -> MatrixMultiply4/1  "C"
  MATLAB Function1/1(S) -> MatrixMultiply/3, MatrixMultiply4/2  "S"
  MATLAB Function8/1(G) -> Add2/3  "G"
  MATLAB Function9/1(S) -> Transpose/1  "S"
  nu/1 -> MatrixMultiply3/3, MatrixMultiply4/3, get nu_acc/1  "v avanz thetadot phidot"
  Transpose/1 -> MatrixMultiply/1, MatrixMultiply2/1
  pid/1 -> MatrixMultiply1/2

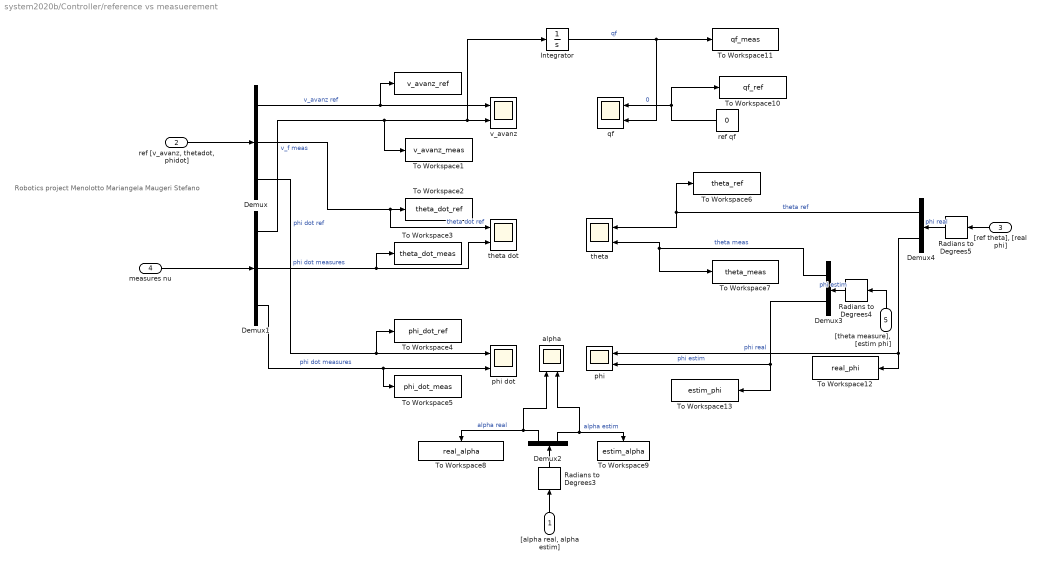
== system system2020b/Controller/reference vs measuerement ==
  note: Robotics project
      | Menolotto Mariangela
      | Maugeri Stefano
  "[alpha real, alpha estim]" : Inport
  "ref [v_avanz, thetadot, phidot]" : Inport  Port=2
  "[ref theta], [real phi]" : Inport  Port=3
  measures nu : Inport  Port=4
  "[theta measure], [estim phi]" : Inport  Port=5
  " " : ToWorkspace  VariableName=v_avanz_ref  SaveFormat=Timeseries  SampleTime=TsGraph
  Demux : Demux  Outputs=3
  Demux1 : Demux  Outputs=3
  Demux2 : Demux  Outputs=2
  Demux3 : Demux  Outputs=2
  Demux4 : Demux  Outputs=2
  Integrator : Integrator
  Radians to Degrees3 : simulink_extras/Transformations/Radians to Degrees
  Radians to Degrees4 : simulink_extras/Transformations/Radians to Degrees
  Radians to Degrees5 : simulink_extras/Transformations/Radians to Degrees
  To Workspace1 : ToWorkspace  VariableName=v_avanz_meas  SaveFormat=Timeseries  SampleTime=TsGraph
  To Workspace10 : ToWorkspace  VariableName=qf_ref  SaveFormat=Timeseries  SampleTime=TsGraph
  To Workspace11 : ToWorkspace  VariableName=qf_meas  SaveFormat=Timeseries  SampleTime=TsGraph
  To Workspace12 : ToWorkspace  VariableName=real_phi  SaveFormat=Timeseries  SampleTime=TsGraph
  To Workspace13 : ToWorkspace  VariableName=estim_phi  SaveFormat=Timeseries  SampleTime=TsGraph
  To Workspace2 : ToWorkspace  VariableName=theta_dot_ref  SaveFormat=Timeseries  SampleTime=TsGraph
  To Workspace3 : ToWorkspace  VariableName=theta_dot_meas  SaveFormat=Timeseries  SampleTime=TsGraph
  To Workspace4 : ToWorkspace  VariableName=phi_dot_ref  SaveFormat=Timeseries  SampleTime=TsGraph
  To Workspace5 : ToWorkspace  VariableName=phi_dot_meas  SaveFormat=Timeseries  SampleTime=TsGraph
  To Workspace6 : ToWorkspace  VariableName=theta_ref  SaveFormat=Timeseries  SampleTime=TsGraph
  To Workspace7 : ToWorkspace  VariableName=theta_meas  SaveFormat=Timeseries  SampleTime=TsGraph
  To Workspace8 : ToWorkspace  VariableName=real_alpha  SaveFormat=Timeseries  SampleTime=TsGraph
  To Workspace9 : ToWorkspace  VariableName=estim_alpha  SaveFormat=Timeseries  SampleTime=TsGraph
  alpha : Scope  NumInputPorts=2
  phi : Scope  NumInputPorts=2
  phi dot : Scope  NumInputPorts=2
  qf : Scope  NumInputPorts=2
  ref qf : Constant  Value=0
  theta : Scope  NumInputPorts=2
  theta dot : Scope  NumInputPorts=2
  v_avanz : Scope  NumInputPorts=2
  wires:
  "ref [v_avanz, thetadot, phidot]"/1 -> Demux/1
  measures nu/1 -> Demux1/1
  Demux/1 -> v_avanz/1, " "/1  "v_avanz ref"
  Demux1/1 -> Integrator/1, v_avanz/2, To Workspace1/1  "v_f meas"
  Demux/2 -> To Workspace2/1, theta dot/1  "theta dot ref"
  Demux1/2 -> theta dot/2, To Workspace3/1  "phi dot measures"
  Demux/3 -> phi dot/1, To Workspace4/1  "phi dot ref"
  Demux1/3 -> To Workspace5/1, phi dot/2  "phi dot measures"
  "[ref theta], [real phi]"/1 -> Radians to Degrees5/1
  "[theta measure], [estim phi]"/1 -> Radians to Degrees4/1
  ref qf/1 -> To Workspace10/1, qf/1  "0"
  Integrator/1 -> qf/2, To Workspace11/1  "qf"
  "[alpha real, alpha estim]"/1 -> Radians to Degrees3/1
  Demux2/1 -> alpha/1, To Workspace8/1  "alpha real"
  Demux2/2 -> To Workspace9/1, alpha/2  "alpha estim"
  Demux3/1 -> To Workspace7/1, theta/2  "theta meas"
  Demux3/2 -> To Workspace13/1, phi/2  "phi estim"
  Demux4/1 -> To Workspace6/1, theta/1  "theta ref"
  Demux4/2 -> phi/1, To Workspace12/1  "phi real"
  Radians to Degrees5/1 -> Demux4/1  "phi real"
  Radians to Degrees4/1 -> Demux3/1  "phi estim"
  Radians to Degrees3/1 -> Demux2/1

== system system2020b/Filtering/Kalman filter ==
  note: Robotics project
      | Menolotto Mariangela
      | Maugeri Stefano
  "[thetar, thetal] meas" : Inport
  v forward : Inport  Port=2
  "[accX, accY, accZ] with noise" : Inport  Port=3
  omega_c : Inport  Port=4
  magnetometer : Inport  Port=5
  Delay : Delay  DelayLength=1  InitialCondition=x0  SampleTime=Ts
  Delay1 : Delay  DelayLength=1  InitialCondition=P0  SampleTime=Ts
  EKF : MATLAB Function  TreatAsAtomicUnit=on
  Mux : Mux  Inputs=3
  store on workspace : Subsystem
  "[v_forward, thetadot, phidot] est" : Outport
  "[alpha theta phi] est" : Outport  Port=2
  wires:
  Mux/1 -> store on workspace/1("[v_avanz real, thetadot, phidot] est"), "[v_forward, thetadot, phidot] est"/1
  EKF/3(angles) -> store on workspace/2("[alpha, theta, phi] est"), "[alpha theta phi] est"/1
  v forward/1 -> Mux/1  "vf"
  EKF/1(theta_dot) -> Mux/2
  EKF/2(phi_dot) -> Mux/3
  "[accX, accY, accZ] with noise"/1 -> EKF/2(acc)
  omega_c/1 -> EKF/3(gyro)
  Delay/1 -> EKF/5("x ")
  EKF/4(x) -> Delay/1
  EKF/5(P) -> Delay1/1
  Delay1/1 -> EKF/6("P ")
  magnetometer/1 -> EKF/4(magn)
  "[thetar, thetal] meas"/1 -> EKF/1(theta_wheels)

== system system2020b/Filtering/Mahony + distance sensor ==
  note: get phi
  note: [v_avanz real, thetadot, phidot] est
  note: get phi dot
  note: Robotics project
      | Menolotto Mariangela
      | Maugeri Stefano
  d : Inport
  "[accX, accY, accZ] with noise" : Inport  Port=2
  omega_c : Inport  Port=3
  magnetomiter : Inport  Port=4
  v forward : Inport  Port=5
  MATLAB Function : MATLAB Function  TreatAsAtomicUnit=on
  Mux1 : Mux  Inputs=3
  Selector : Selector  InputPortWidth=3  IndexOptions=Index vector (dialog)  Indices=3  OutputSizes=1
  get phi from distance sensor : MATLAB Function  TreatAsAtomicUnit=on
  mahony  with quaternions : Subsystem  Commented=on
  mahony filter : Subsystem
  store on workspace : Subsystem
  "[v_avanz real, thetadot, phidot] est" : Outport
  "[alpha theta phi] est" : Outport  Port=2
  wires:
  get phi from distance sensor/1(phi_star) -> mahony filter/1(phi_star)
  Selector/1 -> MATLAB Function/2(phi)  "phi"
  MATLAB Function/2(phidot) -> Mux1/3
  omega_c/1 -> MATLAB Function/1(omega_c), mahony filter/3(omega_c hat with noise)
  d/1 -> get phi from distance sensor/1(d)
  mahony filter/1("[alpha, theta, phi] est") -> "[alpha theta phi] est"/1, store on workspace/2("[alpha, theta, phi] est"), Selector/1  "[alpha theta phi] est and filtered"
  "[accX, accY, accZ] with noise"/1 -> mahony filter/2("[accX, accY, accZ]")
  MATLAB Function/1(thetadot) -> Mux1/2  "theta dot"
  v forward/1 -> Mux1/1
  magnetomiter/1 -> mahony filter/4(magnetometro)
  Mux1/1 -> "[v_avanz real, thetadot, phidot] est"/1, store on workspace/1("[v_avanz real, thetadot, phidot] est")

== system system2020b/Filtering/mux signals ==
  note: Robotics project
      | Menolotto Mariangela
      | Maugeri Stefano
  "[q; nu; q_dot] real" : Inport
  Selector : Selector  InputPortWidth=15  IndexOptions=Index vector (dialog)  Indices=7  OutputSizes=1
  Selector1 : Selector  InputPortWidth=15  IndexOptions=Index vector (dialog)  Indices=[1:9]  OutputSizes=1
  Zero-Order Hold3 : ZeroOrderHold  SampleTime=Ts
  v_forward : Outport
  "[q;nu]" : Outport  Port=2
  wires:
  "[q; nu; q_dot] real"/1 -> Selector1/1, Selector/1
  Selector/1 -> Zero-Order Hold3/1  "v_forward"
  Selector1/1 -> "[q;nu]"/1  "[q;nu]"
  Zero-Order Hold3/1 -> v_forward/1

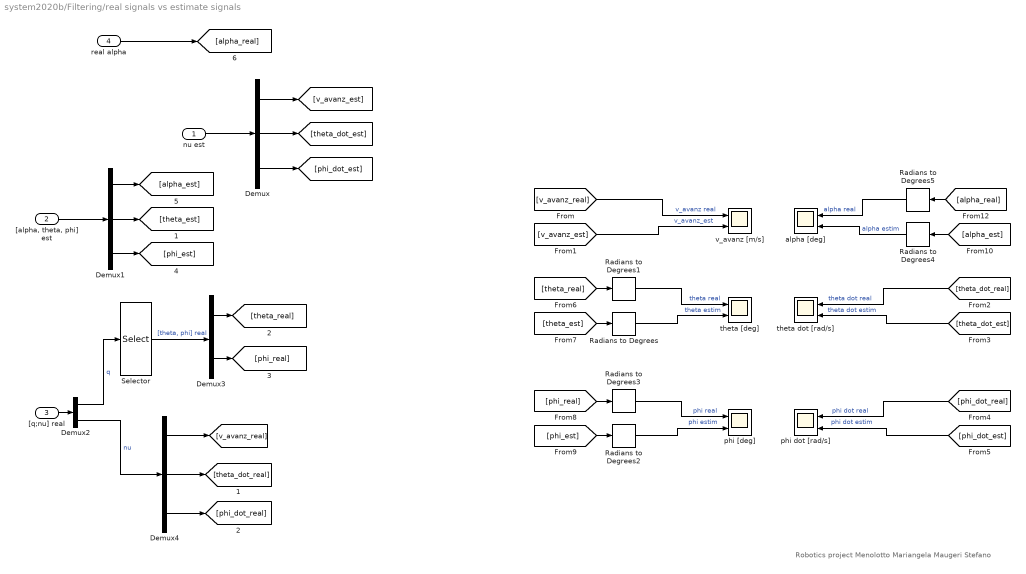
== system system2020b/Filtering/real signals vs estimate signals ==
  note: Robotics project
      | Menolotto Mariangela
      | Maugeri Stefano
  nu est : Inport
  "[alpha, theta, phi] est" : Inport  Port=2
  "[q;nu] real" : Inport  Port=3
  real alpha : Inport  Port=4
  Demux : Demux  Outputs=3
  Demux1 : Demux  Outputs=3
  Demux2 : Demux  Outputs=[6,3]
  Demux3 : Demux  Outputs=2
  Demux4 : Demux  Outputs=3
  Radians to Degrees{,1..5} (6 alike) : simulink_extras/Transformations/Radians to Degrees
  Selector : Selector  InputPortWidth=6  IndexOptions=Index vector (dialog)  Indices=[3 4]  OutputSizes=1
  alpha [deg] : Scope  NumInputPorts=2
  phi [deg] : Scope  NumInputPorts=2
  phi dot [rad/s] : Scope  NumInputPorts=2
  theta [deg] : Scope  NumInputPorts=2
  theta dot [rad/s] : Scope  NumInputPorts=2
  v_avanz [m/s] : Scope  NumInputPorts=2
  wires:
  nu est/1 -> Demux/1
  "[alpha, theta, phi] est"/1 -> Demux1/1
  "[q;nu] real"/1 -> Demux2/1
  Demux2/1 -> Selector/1  "q"
  Selector/1 -> Demux3/1  "[theta, phi] real"
  Demux2/2 -> Demux4/1  "nu"
  Demux4/1 -> [v_avanz_real]
  [v_avanz_real] -> v_avanz [m/s]/1  "v_avanz real"
  Demux/1 -> [v_avanz_est]
  [v_avanz_est] -> v_avanz [m/s]/2  "v_avanz_est"
  [theta_dot_real] -> theta dot [rad/s]/1  "theta dot real"
  [theta_dot_est] -> theta dot [rad/s]/2  "theta dot estim"
  [phi_dot_real] -> phi dot [rad/s]/1  "phi dot real"
  [phi_dot_est] -> phi dot [rad/s]/2  "phi dot estim"
  Demux/2 -> [theta_dot_est]
  Demux/3 -> [phi_dot_est]
  Demux4/2 -> [theta_dot_real]
  Demux4/3 -> [phi_dot_real]
  [theta_est] -> Radians to Degrees/1
  [theta_real] -> Radians to Degrees1/1
  Radians to Degrees/1 -> theta [deg]/2  "theta estim"
  Radians to Degrees1/1 -> theta [deg]/1  "theta real"
  Demux1/2 -> [theta_est]
  Demux3/1 -> [theta_real]
  Radians to Degrees3/1 -> phi [deg]/1  "phi real"
  [phi_real] -> Radians to Degrees3/1
  [phi_est] -> Radians to Degrees2/1
  Radians to Degrees2/1 -> phi [deg]/2  "phi estim"
  Demux3/2 -> [phi_real]
  Demux1/3 -> [phi_est]
  Demux1/1 -> [alpha_est]
  real alpha/1 -> [alpha_real]
  Radians to Degrees4/1 -> alpha [deg]/2  "alpha estim"
  [alpha_real] -> Radians to Degrees5/1
  Radians to Degrees5/1 -> alpha [deg]/1  "alpha real"
  [alpha_est] -> Radians to Degrees4/1

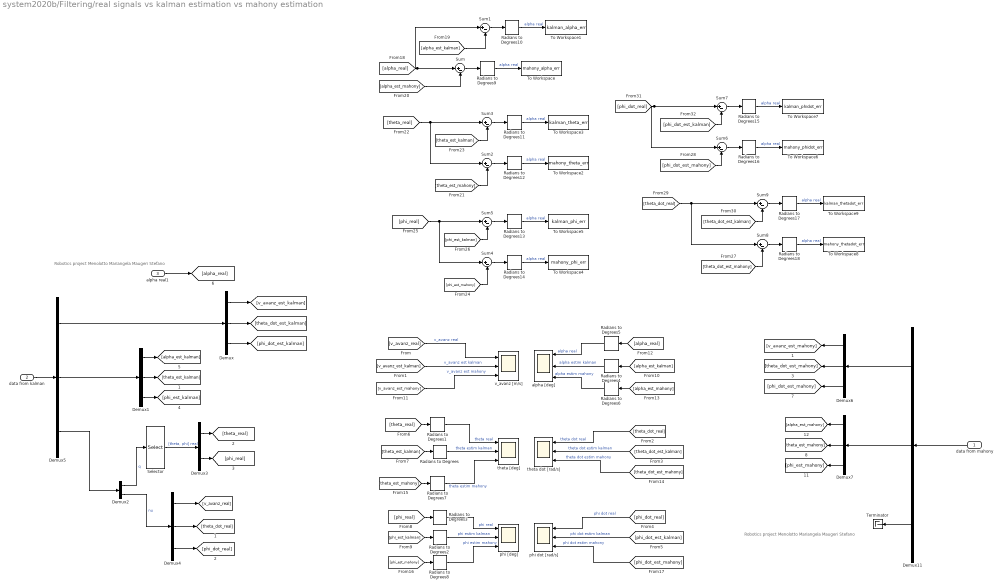
== system system2020b/Filtering/real signals vs kalman estimation vs mahony estimation ==
  note: Robotics project
      | Menolotto Mariangela
      | Maugeri Stefano
  note: Robotics project
      | Menolotto Mariangela
      | Maugeri Stefano
  data from mahony : Inport
  data from kalman : Inport  Port=2
  alpha real1 : Inport  Port=3
  Demux{,1,4,6..7} (5 alike) : Demux  Outputs=3
  Demux11 : Demux  Outputs=[3, 3, 9]
  Demux2 : Demux  Outputs=[6,3]
  Demux3 : Demux  Outputs=2
  Demux5 : Demux  Outputs=[3, 3, 9]
  Radians to Degrees{,1..18} (19 alike) : simulink_extras/Transformations/Radians to Degrees
  Selector : Selector  InputPortWidth=6  IndexOptions=Index vector (dialog)  Indices=[3 4]  OutputSizes=1
  Sum{,1..9} (10 alike) : Sum  Inputs=|+-
  Terminator : Terminator
  To Workspace : ToWorkspace  VariableName=mahony_alpha_err  SaveFormat=Timeseries  SampleTime=Ts
  To Workspace1 : ToWorkspace  VariableName=kalman_alpha_err  SaveFormat=Timeseries  SampleTime=Ts
  To Workspace2 : ToWorkspace  VariableName=mahony_theta_err  SaveFormat=Timeseries  SampleTime=Ts
  To Workspace3 : ToWorkspace  VariableName=kalman_theta_err  SaveFormat=Timeseries  SampleTime=Ts
  To Workspace4 : ToWorkspace  VariableName=mahony_phi_err  SaveFormat=Timeseries  SampleTime=Ts
  To Workspace5 : ToWorkspace  VariableName=kalman_phi_err  SaveFormat=Timeseries  SampleTime=Ts
  To Workspace6 : ToWorkspace  VariableName=mahony_phidot_err  SaveFormat=Timeseries  SampleTime=Ts
  To Workspace7 : ToWorkspace  VariableName=kalman_phidot_err  SaveFormat=Timeseries  SampleTime=Ts
  To Workspace8 : ToWorkspace  VariableName=mahony_thetadot_err  SaveFormat=Timeseries  SampleTime=Ts
  To Workspace9 : ToWorkspace  VariableName=kalman_thetadot_err  SaveFormat=Timeseries  SampleTime=Ts
  alpha [deg] : Scope  NumInputPorts=3
  phi [deg] : Scope  NumInputPorts=3
  phi dot [rad/s] : Scope  NumInputPorts=3
  theta [deg] : Scope  NumInputPorts=3
  theta dot [rad/s] : Scope  NumInputPorts=3
  v_avanz [m/s] : Scope  NumInputPorts=3
  wires:
  [alpha_est_kalman] -> Radians to Degrees4/1
  Radians to Degrees5/1 -> alpha [deg]/1  "alpha real"
  [alpha_real] -> Radians to Degrees5/1
  Radians to Degrees4/1 -> alpha [deg]/2  "alpha estim kalman"
  Demux1/1 -> [alpha_est_kalman]
  Demux1/3 -> [phi_est_kalman]
  Demux3/2 -> [phi_real]
  Radians to Degrees2/1 -> phi [deg]/2  "phi estim kalman"
  [phi_est_kalman] -> Radians to Degrees2/1
  [phi_real] -> Radians to Degrees3/1
  Radians to Degrees3/1 -> phi [deg]/1  "phi real"
  Demux3/1 -> [theta_real]
  Demux1/2 -> [theta_est_kalman]
  Radians to Degrees1/1 -> theta [deg]/1  "theta real"
  Radians to Degrees/1 -> theta [deg]/2  "theta estim kalman"
  [theta_real] -> Radians to Degrees1/1
  [theta_est_kalman] -> Radians to Degrees/1
  Demux4/3 -> [phi_dot_real]
  Demux4/2 -> [theta_dot_real]
  Demux/3 -> [phi_dot_est_kalman]
  Demux/2 -> [theta_dot_est_kalman]
  [phi_dot_est_kalman] -> phi dot [rad/s]/2  "phi dot estim kalman"
  [phi_dot_real] -> phi dot [rad/s]/1  "phi dot real"
  [theta_dot_est_kalman] -> theta dot [rad/s]/2  "theta dot estim kalman"
  [theta_dot_real] -> theta dot [rad/s]/1  "theta dot real"
  [v_avanz_est_kalman] -> v_avanz [m/s]/2  "v_avanz est kalman"
  Demux/1 -> [v_avanz_est_kalman]
  [v_avanz_real] -> v_avanz [m/s]/1  "v_avanz real"
  Demux4/1 -> [v_avanz_real]
  Demux2/2 -> Demux4/1  "nu"
  Selector/1 -> Demux3/1  "[theta, phi] real"
  Demux2/1 -> Selector/1  "q"
  Demux5/3 -> Demux2/1
  Demux5/2 -> Demux1/1
  Demux5/1 -> Demux/1
  data from kalman/1 -> Demux5/1
  alpha real1/1 -> [alpha_real]
  Demux11/2 -> Demux7/1
  data from mahony/1 -> Demux11/1
  Demux6/3 -> [phi_dot_est_mahony]
  Demux7/1 -> [alpha_est_mahony]
  Demux6/2 -> [theta_dot_est_mahony]
  Demux6/1 -> [v_avanz_est_mahony]
  Demux7/3 -> [phi_est_mahony]
  Demux7/2 -> [theta_est_mahony]
  Demux11/1 -> Demux6/1
  Demux11/3 -> Terminator/1
  [v_avanz_est_mahony] -> v_avanz [m/s]/3  "v_avanz est mahony"
  [alpha_est_mahony] -> Radians to Degrees6/1
  Radians to Degrees6/1 -> alpha [deg]/3  "alpha estim mahony"
  [theta_dot_est_mahony] -> theta dot [rad/s]/3  "theta dot estim mahony"
  [theta_est_mahony] -> Radians to Degrees7/1
  Radians to Degrees7/1 -> theta [deg]/3  "theta estim mahony"
  [phi_est_mahony] -> Radians to Degrees8/1
  Radians to Degrees8/1 -> phi [deg]/3  "phi estim mahony"
  [phi_dot_est_mahony] -> phi dot [rad/s]/3  "phi dot estim mahony"
  Radians to Degrees16/1 -> To Workspace6/1  "alpha real"
  Radians to Degrees15/1 -> To Workspace7/1  "alpha real"
  [theta_real] -> Sum2/1, Sum3/1
  [phi_dot_est_mahony] -> Sum6/2
  [alpha_est_mahony] -> Sum/2
  [theta_est_kalman] -> Sum3/2
  Radians to Degrees9/1 -> To Workspace/1  "alpha real"
  [theta_est_mahony] -> Sum2/2
  [theta_dot_est_kalman] -> Sum9/2
  [alpha_est_kalman] -> Sum1/2
  Radians to Degrees14/1 -> To Workspace4/1  "alpha real"
  Radians to Degrees10/1 -> To Workspace1/1  "alpha real"
  Radians to Degrees13/1 -> To Workspace5/1  "alpha real"
  [phi_dot_est_kalman] -> Sum7/2
  Sum4/1 -> Radians to Degrees14/1
  Radians to Degrees18/1 -> To Workspace8/1  "alpha real"
  Sum5/1 -> Radians to Degrees13/1
  [phi_dot_real] -> Sum7/1, Sum6/1
  Sum6/1 -> Radians to Degrees16/1
  Sum/1 -> Radians to Degrees9/1
  Sum1/1 -> Radians to Degrees10/1
  [alpha_real] -> Sum/1, Sum1/1
  [phi_est_kalman] -> Sum5/2
  [phi_est_mahony] -> Sum4/2
  [theta_dot_real] -> Sum9/1, Sum8/1
  Radians to Degrees12/1 -> To Workspace2/1  "alpha real"
  Sum2/1 -> Radians to Degrees12/1
  Sum3/1 -> Radians to Degrees11/1
  Radians to Degrees11/1 -> To Workspace3/1  "alpha real"
  Sum7/1 -> Radians to Degrees15/1
  Sum8/1 -> Radians to Degrees18/1
  [theta_dot_est_mahony] -> Sum8/2
  Sum9/1 -> Radians to Degrees17/1
  Radians to Degrees17/1 -> To Workspace9/1  "alpha real"
  [phi_real] -> Sum5/1, Sum4/1

== system system2020b/Physical system/old model ==
  note: Robotics project
      | Menolotto Mariangela
      | Maugeri Stefano
  " " : ManualSwitch  CurrentSetting=0
  Constant1 : Constant  Value=[0;0]
  LQR con linearizzato : Subsystem
  Scope4 : Scope
  Scope5 : Scope
  Sistema fisico1 : Subsystem
  deg1 : Display
  wires:
  LQR con linearizzato/1(tau) -> " "/2
  Sistema fisico1/2(alpha (deg)) -> deg1/1
  Constant1/1 -> " "/1
  " "/1 -> Sistema fisico1/1(tau)
  Sistema fisico1/3(nu) -> LQR con linearizzato/2(nu), Scope5/1  "[nu1,nu2,nu3] -> [vavanz, thetadot, phidot]"
  Sistema fisico1/1(q) -> LQR con linearizzato/1(q), Scope4/1  "[x,y,theta,phi,thetar,thetal]"

== system system2020b/Reference generator/manual ==
  note: Robotics project
      | Menolotto Mariangela
      | Maugeri Stefano
  CONTROLLO POSIZIONE : Constant  Value=2
  CONTROLLO VELOCITA' : Constant
  Manual Switch1 : ManualSwitch
  Mux : Mux
  alpha : Constant  Value=0
  theta : Constant  Value=90
  v_avanz : Constant  Value=0
  "[control_type, v_avanz, theta, alpha]" : Outport
  wires:
  v_avanz/1 -> Mux/2  "v_avanz m/s"
  theta/1 -> Mux/3  "theta deg"
  alpha/1 -> Mux/4  "alpha in deg"
  Manual Switch1/1 -> Mux/1  "controlType [1/2]"
  Mux/1 -> "[control_type, v_avanz, theta, alpha]"/1
  CONTROLLO VELOCITA'/1 -> Manual Switch1/1
  CONTROLLO POSIZIONE/1 -> Manual Switch1/2

== system system2020b/Reference generator/ref 1, id 2 ==
  note: Robotics project
      | Menolotto Mariangela
      | Maugeri Stefano
  Clock : Clock
  MATLAB Function : MATLAB Function  TreatAsAtomicUnit=on
  Mux : Mux
  "[control_type, v_avanz, theta, alpha]" : Outport
  wires:
  Mux/1 -> "[control_type, v_avanz, theta, alpha]"/1
  MATLAB Function/1(control_type) -> Mux/1  "controlType"
  MATLAB Function/4(alpha) -> Mux/4  "alpha in deg"
  MATLAB Function/3(theta_ref) -> Mux/3  "theta_ref"
  Clock/1 -> MATLAB Function/1(time)
  MATLAB Function/2(v_avanz) -> Mux/2  "v_avanz"

== system system2020b/Reference generator/ref 2, id 3 ==
  note: Robotics project
      | Menolotto Mariangela
      | Maugeri Stefano
  Clock : Clock
  MATLAB Function : MATLAB Function  TreatAsAtomicUnit=on
  Mux : Mux
  "[control_type, v_avanz, theta, alpha]" : Outport
  wires:
  Mux/1 -> "[control_type, v_avanz, theta, alpha]"/1
  MATLAB Function/1(control_type) -> Mux/1  "controlType"
  MATLAB Function/4(alpha) -> Mux/4  "alpha in deg"
  MATLAB Function/3(theta_ref) -> Mux/3  "theta_ref"
  Clock/1 -> MATLAB Function/1(time)
  MATLAB Function/2(v_avanz) -> Mux/2  "v_avanz"

== system system2020b/Reference generator/ref 3, id 4 ==
  note: Robotics project
      | Menolotto Mariangela
      | Maugeri Stefano
  Clock : Clock
  MATLAB Function : MATLAB Function  TreatAsAtomicUnit=on
  Mux : Mux
  "[control_type, v_avanz, theta, alpha]" : Outport
  wires:
  Mux/1 -> "[control_type, v_avanz, theta, alpha]"/1
  MATLAB Function/1(control_type) -> Mux/1  "controlType"
  MATLAB Function/4(alpha) -> Mux/4  "alpha in deg"
  MATLAB Function/3(theta_ref) -> Mux/3  "theta_ref"
  Clock/1 -> MATLAB Function/1(time)
  MATLAB Function/2(v_avanz) -> Mux/2  "v_avanz"

== system system2020b/Reference generator/ref 4, id 5 ==
  note: Robotics project
      | Menolotto Mariangela
      | Maugeri Stefano
  Clock : Clock
  MATLAB Function : MATLAB Function  TreatAsAtomicUnit=on
  Mux : Mux
  "[control_type, v_avanz, theta, alpha]" : Outport
  wires:
  MATLAB Function/2(v_avanz) -> Mux/2  "v_avanz"
  Clock/1 -> MATLAB Function/1(time)
  MATLAB Function/3(theta_ref) -> Mux/3  "theta_ref"
  MATLAB Function/4(alpha) -> Mux/4  "alpha in deg"
  MATLAB Function/1(control_type) -> Mux/1  "controlType"
  Mux/1 -> "[control_type, v_avanz, theta, alpha]"/1

== system system2020b/Reference generator/ref 5, id 6 ==
  note: Robotics project
      | Menolotto Mariangela
      | Maugeri Stefano
  Clock : Clock
  MATLAB Function : MATLAB Function  TreatAsAtomicUnit=on
  Mux : Mux
  "[control_type, v_avanz, theta, alpha]" : Outport
  wires:
  Mux/1 -> "[control_type, v_avanz, theta, alpha]"/1
  MATLAB Function/1(control_type) -> Mux/1  "controlType"
  MATLAB Function/4(alpha) -> Mux/4  "alpha in deg"
  MATLAB Function/3(theta_ref) -> Mux/3  "theta_ref"
  Clock/1 -> MATLAB Function/1(time)
  MATLAB Function/2(v_avanz) -> Mux/2  "v_avanz"

== system system2020b/Reference generator/ref 6, id 7 ==
  note: Robotics project
      | Menolotto Mariangela
      | Maugeri Stefano
  Clock : Clock
  MATLAB Function : MATLAB Function  TreatAsAtomicUnit=on
  Mux : Mux
  "[control_type, v_avanz, theta, alpha]" : Outport
  wires:
  MATLAB Function/2(v_avanz) -> Mux/2  "v_avanz"
  Clock/1 -> MATLAB Function/1(time)
  MATLAB Function/3(theta_ref) -> Mux/3  "theta_ref"
  MATLAB Function/4(alpha) -> Mux/4  "alpha in deg"
  MATLAB Function/1(control_type) -> Mux/1  "controlType"
  Mux/1 -> "[control_type, v_avanz, theta, alpha]"/1

== system system2020b/Reference generator/ref 7, id 8 ==
  note: Robotics project
      | Menolotto Mariangela
      | Maugeri Stefano
  Clock : Clock
  MATLAB Function : MATLAB Function  TreatAsAtomicUnit=on
  Mux : Mux
  "[control_type, v_avanz, theta, alpha]" : Outport
  wires:
  Mux/1 -> "[control_type, v_avanz, theta, alpha]"/1
  MATLAB Function/1(control_type) -> Mux/1  "controlType"
  MATLAB Function/4(alpha) -> Mux/4  "alpha in deg"
  MATLAB Function/3(theta_ref) -> Mux/3  "theta_ref"
  Clock/1 -> MATLAB Function/1(time)
  MATLAB Function/2(v_avanz) -> Mux/2  "v_avanz"

== system system2020b/Reference generator/ref 8, id 9 ==
  note: Robotics project
      | Menolotto Mariangela
      | Maugeri Stefano
  Clock : Clock
  MATLAB Function1 : MATLAB Function  TreatAsAtomicUnit=on
  MATLAB Function2 : MATLAB Function  Commented=on  TreatAsAtomicUnit=on
  Mux : Mux
  XY Graph : simulink/Sinks/XY Graph  Commented=on  xmin=-5  xmax=5  ymin=-5  ymax=5  st=-1
  "[control_type, v_avanz, theta, alpha]" : Outport
  wires:
  MATLAB Function1/2(v_avanz) -> Mux/2  "v_avanz"
  Clock/1 -> MATLAB Function1/1(time)
  MATLAB Function1/3(theta) -> Mux/3  "theta_ref"
  MATLAB Function1/4(alpha) -> Mux/4  "alpha in deg"
  MATLAB Function1/1(control_type) -> Mux/1  "controlType"
  Mux/1 -> "[control_type, v_avanz, theta, alpha]"/1

== system system2020b/Reference generator/ref 9, id 10 ==
  note: Robotics project
      | Menolotto Mariangela
      | Maugeri Stefano
  Clock : Clock
  MATLAB Function : MATLAB Function  TreatAsAtomicUnit=on
  Mux : Mux
  Zero-Order Hold1 : ZeroOrderHold  SampleTime=Ts
  "[control_type, v_avanz, theta, alpha]" : Outport
  wires:
  Mux/1 -> "[control_type, v_avanz, theta, alpha]"/1
  MATLAB Function/1(control_type) -> Mux/1  "controlType"
  MATLAB Function/4(alpha) -> Mux/4  "alpha in deg"
  MATLAB Function/3(theta) -> Mux/3  "theta_ref"
  Clock/1 -> Zero-Order Hold1/1
  MATLAB Function/2(v_avanz) -> Mux/2  "v_avanz"
  Zero-Order Hold1/1 -> MATLAB Function/1(time)
